simulink model "Motor_Fault_System"  (R2025b)
settings: Solver=ode4  StartTime=0.0  StopTime=30  FixedStep=0.01  RelTol=1e-3
settings Model: Creator=anifa  LastModifiedBy=anifa

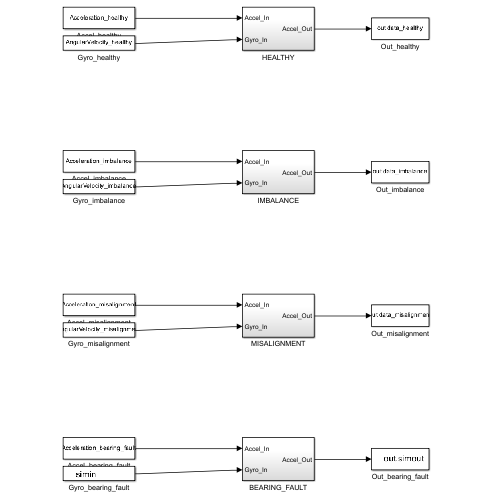
[thumbnail: Simulink's stored preview of the top-level diagram]
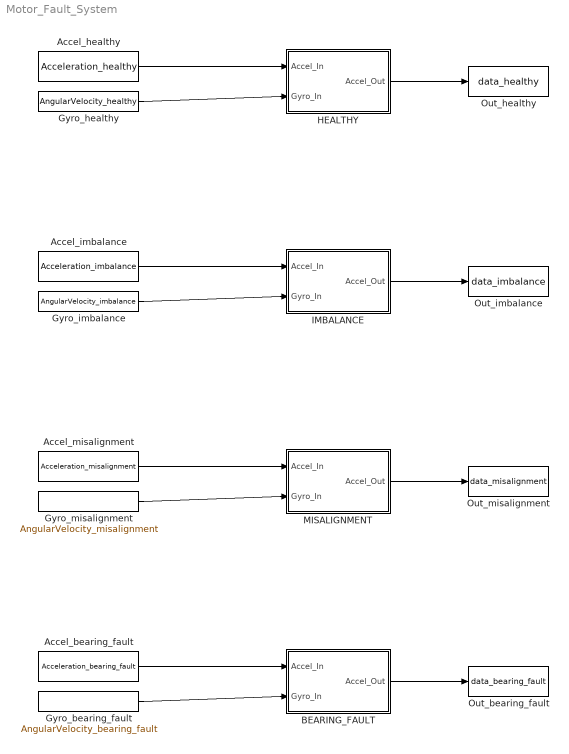
== system Motor_Fault_System ==
  Accel_bearing_fault : FromWorkspace  VariableName=Acceleration_bearing_fault
  Accel_healthy : FromWorkspace  VariableName=Acceleration_healthy
  Accel_imbalance : FromWorkspace  VariableName=Acceleration_imbalance
  Accel_misalignment : FromWorkspace  VariableName=Acceleration_misalignment
  BEARING_FAULT : Subsystem
  Gyro_bearing_fault : FromWorkspace  VariableName=AngularVelocity_bearing_fault
  Gyro_healthy : FromWorkspace  VariableName=AngularVelocity_healthy
  Gyro_imbalance : FromWorkspace  VariableName=AngularVelocity_imbalance
  Gyro_misalignment : FromWorkspace  VariableName=AngularVelocity_misalignment
  HEALTHY : Subsystem
  IMBALANCE : Subsystem
  MISALIGNMENT : Subsystem
  Out_bearing_fault : ToWorkspace  VariableName=data_bearing_fault  SaveFormat=Timeseries  SampleTime=-1
  Out_healthy : ToWorkspace  VariableName=data_healthy  SaveFormat=Timeseries  SampleTime=-1
  Out_imbalance : ToWorkspace  VariableName=data_imbalance  SaveFormat=Timeseries  SampleTime=-1
  Out_misalignment : ToWorkspace  VariableName=data_misalignment  SaveFormat=Timeseries  SampleTime=-1
  wires:
  Accel_healthy/1 -> HEALTHY/1(Accel_In)
  Gyro_healthy/1 -> HEALTHY/2(Gyro_In)
  HEALTHY/1(Accel_Out) -> Out_healthy/1
  Accel_imbalance/1 -> IMBALANCE/1(Accel_In)
  Gyro_imbalance/1 -> IMBALANCE/2(Gyro_In)
  IMBALANCE/1(Accel_Out) -> Out_imbalance/1
  Accel_misalignment/1 -> MISALIGNMENT/1(Accel_In)
  Gyro_misalignment/1 -> MISALIGNMENT/2(Gyro_In)
  MISALIGNMENT/1(Accel_Out) -> Out_misalignment/1
  Accel_bearing_fault/1 -> BEARING_FAULT/1(Accel_In)
  Gyro_bearing_fault/1 -> BEARING_FAULT/2(Gyro_In)
  BEARING_FAULT/1(Accel_Out) -> Out_bearing_fault/1

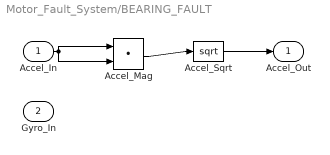
== system Motor_Fault_System/BEARING_FAULT ==
  Accel_In : Inport
  Gyro_In : Inport  Port=2
  Accel_Mag : DotProduct  OutDataTypeStr=Inherit: Inherit via internal rule
  Accel_Sqrt : Sqrt
  Accel_Out : Outport
  wires:
  Accel_In/1 -> Accel_Mag/1, Accel_Mag/2
  Accel_Mag/1 -> Accel_Sqrt/1
  Accel_Sqrt/1 -> Accel_Out/1

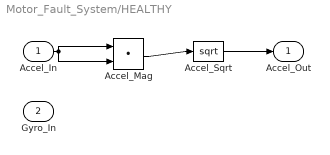
== system Motor_Fault_System/HEALTHY ==
  Accel_In : Inport
  Gyro_In : Inport  Port=2
  Accel_Mag : DotProduct  OutDataTypeStr=Inherit: Inherit via internal rule
  Accel_Sqrt : Sqrt
  Accel_Out : Outport
  wires:
  Accel_In/1 -> Accel_Mag/1, Accel_Mag/2
  Accel_Mag/1 -> Accel_Sqrt/1
  Accel_Sqrt/1 -> Accel_Out/1

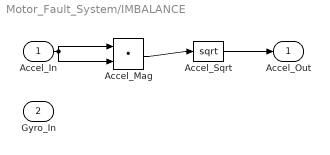
== system Motor_Fault_System/IMBALANCE ==
  Accel_In : Inport
  Gyro_In : Inport  Port=2
  Accel_Mag : DotProduct  OutDataTypeStr=Inherit: Inherit via internal rule
  Accel_Sqrt : Sqrt
  Accel_Out : Outport
  wires:
  Accel_In/1 -> Accel_Mag/1, Accel_Mag/2
  Accel_Mag/1 -> Accel_Sqrt/1
  Accel_Sqrt/1 -> Accel_Out/1

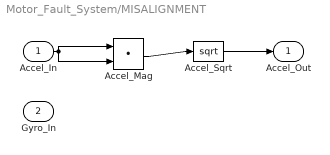
== system Motor_Fault_System/MISALIGNMENT ==
  Accel_In : Inport
  Gyro_In : Inport  Port=2
  Accel_Mag : DotProduct  OutDataTypeStr=Inherit: Inherit via internal rule
  Accel_Sqrt : Sqrt
  Accel_Out : Outport
  wires:
  Accel_In/1 -> Accel_Mag/1, Accel_Mag/2
  Accel_Mag/1 -> Accel_Sqrt/1
  Accel_Sqrt/1 -> Accel_Out/1
